simulink model "mrefrobotarm_modified_previous_y_previous_u_previous_ref_pert_2"  (R2018b)
settings: Solver=FixedStepAuto  StartTime=0.0  StopTime=60  RelTol=1e-3  AbsTol=1e-6
undefined symbols (not defined in the file or in its folder): cc, options
libraries: neural x858, simulink x1
(part 20 of 32)

== system mrefrobotarm_modified_previous_y_previous_u_previous_ref_pert_2/m=0 sd=0.3/Layer 3/Delays 1 ==
  "p{3}" : Inport  PortDimensions=30
      mask Display: e = 0.06;c1 = [120 230 180]/255;c2 = ([120 230 180]+0)/(256+128);c3 = ([120 230 180]+128)/(256+128);patch([0 1 1 0],[0 0 1 1],c1);patch([0 1 1 1-e 1-e 0+e],[0 0 1 1-e 0+e 0+e],c2);patch([0 0 1 1-e 0+e 0+e],[0 1 1 1-e 1-e 0+e],c3);plot([0 1 1 0 0],[0 0 1 1 0]);
  mux : Mux  Inputs=1
      mask Display: e = 0.06;c1 = [120 150 230]/255;c2 = ([120 150 230]+0)/383;c3 = ([120 150 230]+128)/383;patch([0 1 1 0],[0 0 1 1],c1);patch([0 1 1 1-e 1-e 0+e],[0 0 1 1-e 0+e 0+e],c2);patch([0 0 1 1-e 0+e 0+e],[0 1 1 1-e 1-e 0+e],c3);plot([0 1 1 0 0],[0 0 1 1 0]);disp('Mux')
  "pd{3,2}" : Outport
      mask Display: e = 0.06;c1 = [120 230 180]/255;c2 = ([120 230 180]+0)/(256+128);c3 = ([120 230 180]+128)/(256+128);patch([0 1 1 0],[0 0 1 1],c1);patch([0 1 1 1-e 1-e 0+e],[0 0 1 1-e 0+e 0+e],c2);patch([0 0 1 1-e 0+e 0+e],[0 1 1 1-e 1-e 0+e],c3);plot([0 1 1 0 0],[0 0 1 1 0]);
  wires:
  "p{3}"/1 -> mux/1
  mux/1 -> "pd{3,2}"/1

== system mrefrobotarm_modified_previous_y_previous_u_previous_ref_pert_2/m=0 sd=0.3/Layer 3/LW{3,2} ==
  "ad{3,2}" : Inport  PortDimensions=30
      mask Display: e = 0.06;c1 = [120 230 180]/255;c2 = ([120 230 180]+0)/(256+128);c3 = ([120 230 180]+128)/(256+128);patch([0 1 1 0],[0 0 1 1],c1);patch([0 1 1 1-e 1-e 0+e],[0 0 1 1-e 0+e 0+e],c2);patch([0 0 1 1-e 0+e 0+e],[0 1 1 1-e 1-e 0+e],c3);plot([0 1 1 0 0],[0 0 1 1 0]);
  "IW{3,2}(1,:)'" : Constant  Value=[0.00073031899760629269587053347123628554982133209705352783203125;0.00015755393865115070316414158657636335192364640533924102783203125;-0.001153726580471188360721424004395885276608169078826904296875;-0.000147810248176156772310918530166645723511464893817901611328125;-0.0003676237953308994737926240770065078322659246623516082763671875;2.047747561014855666172707060468383133411407470703125;-0.000120078654340241940796062125595966563196270726621150970458984375;-0.0001517146347455816213049828444781041980604641139507293701171875;0.001069066277835455623657079371469080797396600246429443359375;-0.000455869268953239151036249676707257094676606357097625732421875;-0.000131416867977301771337750313506376187433488667011260986328125;0.0021027852077354597208624920057218332658521831035614013671875;-0.000428718552194034228930430430182241252623498439788818359375;0.000668702472228331818750179937893562964745797216892242431640625;-0.0002648472831370911047092764345478599352645687758922576904296875;-0.00225575463499039750858710107195292948745191097259521484375;-9.959793829520429873057574265970970373018644750118255615234375e-05;0.00081342038300134486029924207883823328302241861820220947265625;-0.000264647625776768852419451594215615841676481068134307861328125;0.000243069440059264798258131801134140914655290544033050537109375;0.0002546442972532542343457040434628879665979184210300445556640625;-0.000265938721012887375506894560572845875867642462253570556640625;2.880739455805856856908213348145153531731921248137950897216796875e-05;0.0002520358189922171517592663914086870136088691651821136474609375;0.000356179041941332113867246800253951732884161174297332763671875;-0.00126836362647298286389363486392767299548722803592681884765625;-0.00020884518780916460647077703693952344110584817826747894287109375;-0.00105229721959188590556244502494109838153235614299774169921875;0.00416506829530418308527028870003050542436540126800537109375;-0.000261752708499157099066023679512227317900396883487701416015625]
      mask Display: e = 0.06;c1 = [120 150 230]/255;c2 = ([120 150 230]+0)/383;c3 = ([120 150 230]+128)/383;patch([0 1 1 0],[0 0 1 1],c1);patch([0 1 1 1-e 1-e 0+e],[0 0 1 1-e 0+e 0+e],c2);patch([0 0 1 1-e 0+e 0+e],[0 1 1 1-e 1-e 0+e],c3);plot([0 1 1 0 0],[0 0 1 1 0]);disp('weights');
  Mux : Mux  Inputs=1
      mask Display: e = 0.06;c1 = [120 150 230]/255;c2 = ([120 150 230]+0)/383;c3 = ([120 150 230]+128)/383;patch([0 1 1 0],[0 0 1 1],c1);patch([0 1 1 1-e 1-e 0+e],[0 0 1 1-e 0+e 0+e],c2);patch([0 0 1 1-e 0+e 0+e],[0 1 1 1-e 1-e 0+e],c3);plot([0 1 1 0 0],[0 0 1 1 0]);disp('Mux');
  dotprod1 : neural/Weight Functions/dotprod
  "lz{3,2}" : Outport
      mask Display: e = 0.06;c1 = [120 230 180]/255;c2 = ([120 230 180]+0)/(256+128);c3 = ([120 230 180]+128)/(256+128);patch([0 1 1 0],[0 0 1 1],c1);patch([0 1 1 1-e 1-e 0+e],[0 0 1 1-e 0+e 0+e],c2);patch([0 0 1 1-e 0+e 0+e],[0 1 1 1-e 1-e 0+e],c3);plot([0 1 1 0 0],[0 0 1 1 0]);
  wires:
  "IW{3,2}(1,:)'"/1 -> dotprod1/1
  "ad{3,2}"/1 -> dotprod1/2
  dotprod1/1 -> Mux/1
  Mux/1 -> "lz{3,2}"/1

== system mrefrobotarm_modified_previous_y_previous_u_previous_ref_pert_2/m=0 sd=0.4/Layer 1/Delays 1 ==
  "p{1}" : Inport  PortDimensions=10
      mask Display: e = 0.06;c1 = [120 230 180]/255;c2 = ([120 230 180]+0)/(256+128);c3 = ([120 230 180]+128)/(256+128);patch([0 1 1 0],[0 0 1 1],c1);patch([0 1 1 1-e 1-e 0+e],[0 0 1 1-e 0+e 0+e],c2);patch([0 0 1 1-e 0+e 0+e],[0 1 1 1-e 1-e 0+e],c3);plot([0 1 1 0 0],[0 0 1 1 0]);
  mux : Mux  Inputs=1
      mask Display: e = 0.06;c1 = [120 150 230]/255;c2 = ([120 150 230]+0)/383;c3 = ([120 150 230]+128)/383;patch([0 1 1 0],[0 0 1 1],c1);patch([0 1 1 1-e 1-e 0+e],[0 0 1 1-e 0+e 0+e],c2);patch([0 0 1 1-e 0+e 0+e],[0 1 1 1-e 1-e 0+e],c3);plot([0 1 1 0 0],[0 0 1 1 0]);disp('Mux')
  "pd{1,1}" : Outport
      mask Display: e = 0.06;c1 = [120 230 180]/255;c2 = ([120 230 180]+0)/(256+128);c3 = ([120 230 180]+128)/(256+128);patch([0 1 1 0],[0 0 1 1],c1);patch([0 1 1 1-e 1-e 0+e],[0 0 1 1-e 0+e 0+e],c2);patch([0 0 1 1-e 0+e 0+e],[0 1 1 1-e 1-e 0+e],c3);plot([0 1 1 0 0],[0 0 1 1 0]);
  wires:
  "p{1}"/1 -> mux/1
  mux/1 -> "pd{1,1}"/1

== system mrefrobotarm_modified_previous_y_previous_u_previous_ref_pert_2/m=0 sd=0.4/Layer 1/IW{1,1} ==
  "pd{1,1}" : Inport  PortDimensions=10
      mask Display: e = 0.06;c1 = [120 230 180]/255;c2 = ([120 230 180]+0)/(256+128);c3 = ([120 230 180]+128)/(256+128);patch([0 1 1 0],[0 0 1 1],c1);patch([0 1 1 1-e 1-e 0+e],[0 0 1 1-e 0+e 0+e],c2);patch([0 0 1 1-e 0+e 0+e],[0 1 1 1-e 1-e 0+e],c3);plot([0 1 1 0 0],[0 0 1 1 0]);
  "IW{1,1}(1,:)'" : Constant  Value=[4.35535709086524747135626967065036296844482421875;2.42555138809412351719174694153480231761932373046875;-3.131200533605130065240018666372634470462799072265625;-0.5094204285878898286199500944348983466625213623046875;-4.1124371498059364427035689004696905612945556640625;0.51883527624200365124806921812705695629119873046875;6.2562144583090031346728210337460041046142578125;6.60866111511276432821659909677691757678985595703125;-18.935865072294749467118890606798231601715087890625;-15.8212895515813567470786438207142055034637451171875]
      mask Display: e = 0.06;c1 = [120 150 230]/255;c2 = ([120 150 230]+0)/383;c3 = ([120 150 230]+128)/383;patch([0 1 1 0],[0 0 1 1],c1);patch([0 1 1 1-e 1-e 0+e],[0 0 1 1-e 0+e 0+e],c2);patch([0 0 1 1-e 0+e 0+e],[0 1 1 1-e 1-e 0+e],c3);plot([0 1 1 0 0],[0 0 1 1 0]);disp('Weights');
  "IW{1,1}(10,:)'" : Constant  Value=[0.53661031067499298519152262088027782738208770751953125;-1.5017668136177440008083294742391444742679595947265625;0.7806843435083996585177601446048356592655181884765625;-0.04055167714109038368253123962858808226883411407470703125;0.46745642085633065665462027027388103306293487548828125;-0.2664486916861605880768593124230392277240753173828125;-0.46684646576965327380293047099257819354534149169921875;-0.29181588578157813262947684052051045000553131103515625;0.985643356544671167540627720882184803485870361328125;0.50112926067407881358661825288436375558376312255859375]
      mask Display: e = 0.06;c1 = [120 150 230]/255;c2 = ([120 150 230]+0)/383;c3 = ([120 150 230]+128)/383;patch([0 1 1 0],[0 0 1 1],c1);patch([0 1 1 1-e 1-e 0+e],[0 0 1 1-e 0+e 0+e],c2);patch([0 0 1 1-e 0+e 0+e],[0 1 1 1-e 1-e 0+e],c3);plot([0 1 1 0 0],[0 0 1 1 0]);disp('Weights');
  "IW{1,1}(11,:)'" : Constant  Value=[-1.6208798224016811584391462019993923604488372802734375;0.447427977253705144722317754713003523647785186767578125;0.4326080920180384037365683980169706046581268310546875;-0.35807065114767600011447257202235050499439239501953125;0.1833514237293495108271912386044277809560298919677734375;-0.498128112866548067305672020665952004492282867431640625;-0.475650781956347523671269073020084761083126068115234375;-0.46513054714543067280629884407971985638141632080078125;0.65795479078694996122322891096700914204120635986328125;0.25047233937190338526335153801483102142810821533203125]
      mask Display: e = 0.06;c1 = [120 150 230]/255;c2 = ([120 150 230]+0)/383;c3 = ([120 150 230]+128)/383;patch([0 1 1 0],[0 0 1 1],c1);patch([0 1 1 1-e 1-e 0+e],[0 0 1 1-e 0+e 0+e],c2);patch([0 0 1 1-e 0+e 0+e],[0 1 1 1-e 1-e 0+e],c3);plot([0 1 1 0 0],[0 0 1 1 0]);disp('Weights');
  "IW{1,1}(12,:)'" : Constant  Value=[0.89487420700217013003197052967152558267116546630859375;0.0736102811658177202946973238795180805027484893798828125;-0.72097767859178352178872728472924791276454925537109375;0.343010449570382291994974366389214992523193359375;0.05526766853889926445209113126111333258450031280517578125;0.1617754949706347866733580076470389030873775482177734375;-0.09925881285950004240259403331947396509349346160888671875;-0.09491493432806123731193537196304532699286937713623046875;0.266775373828542938792196537178824655711650848388671875;0.296807590311673086258537068715668283402919769287109375]
      mask Display: e = 0.06;c1 = [120 150 230]/255;c2 = ([120 150 230]+0)/383;c3 = ([120 150 230]+128)/383;patch([0 1 1 0],[0 0 1 1],c1);patch([0 1 1 1-e 1-e 0+e],[0 0 1 1-e 0+e 0+e],c2);patch([0 0 1 1-e 0+e 0+e],[0 1 1 1-e 1-e 0+e],c3);plot([0 1 1 0 0],[0 0 1 1 0]);disp('Weights');
  "IW{1,1}(13,:)'" : Constant  Value=[1.0693210911560055986768702496192418038845062255859375;-0.921086541198619546122472456772811710834503173828125;-0.39419926353010570352353170164860785007476806640625;0.6864400832934258733786236916785128414630889892578125;0.13946629961123024887825749829062260687351226806640625;2.8551210111443499073402563226409256458282470703125;-2.673885338519812915336615333217196166515350341796875;-0.434420113181992195716674132199841551482677459716796875;7.617755568501014096227663685567677021026611328125;6.32093063063102977849894159589894115924835205078125]
      mask Display: e = 0.06;c1 = [120 150 230]/255;c2 = ([120 150 230]+0)/383;c3 = ([120 150 230]+128)/383;patch([0 1 1 0],[0 0 1 1],c1);patch([0 1 1 1-e 1-e 0+e],[0 0 1 1-e 0+e 0+e],c2);patch([0 0 1 1-e 0+e 0+e],[0 1 1 1-e 1-e 0+e],c3);plot([0 1 1 0 0],[0 0 1 1 0]);disp('Weights');
  "IW{1,1}(14,:)'" : Constant  Value=[1.58733266996484001509770678239874541759490966796875;-1.9550364500455401639555930159986019134521484375;1.193738170368206841231994985719211399555206298828125;0.1743957236971513113932275018669315613806247711181640625;-0.495270571163230866051918610537541098892688751220703125;0.86398853547281861953166526291170157492160797119140625;0.6502199929278200674076515497290529310703277587890625;0.88327744406018349199172234875732101500034332275390625;-0.7161113464611228440759305158280767500400543212890625;1.1400929339190881695031976050813682377338409423828125]
      mask Display: e = 0.06;c1 = [120 150 230]/255;c2 = ([120 150 230]+0)/383;c3 = ([120 150 230]+128)/383;patch([0 1 1 0],[0 0 1 1],c1);patch([0 1 1 1-e 1-e 0+e],[0 0 1 1-e 0+e 0+e],c2);patch([0 0 1 1-e 0+e 0+e],[0 1 1 1-e 1-e 0+e],c3);plot([0 1 1 0 0],[0 0 1 1 0]);disp('Weights');
  "IW{1,1}(15,:)'" : Constant  Value=[0.45779947364027151479604071937501430511474609375;0.70223579556577020444052550374181009829044342041015625;-0.1281575453302842004799089181688032113015651702880859375;0.12564794902972320489453750269603915512561798095703125;-0.381645372211093292236228080582804977893829345703125;-0.0204190490741921228112776276475415215827524662017822265625;1.0790025966145158076159304982866160571575164794921875;0.287301338557884256008634338286356069147586822509765625;-2.2765111432902305210745907970704138278961181640625;-0.86693087767997401016373260063119232654571533203125]
      mask Display: e = 0.06;c1 = [120 150 230]/255;c2 = ([120 150 230]+0)/383;c3 = ([120 150 230]+128)/383;patch([0 1 1 0],[0 0 1 1],c1);patch([0 1 1 1-e 1-e 0+e],[0 0 1 1-e 0+e 0+e],c2);patch([0 0 1 1-e 0+e 0+e],[0 1 1 1-e 1-e 0+e],c3);plot([0 1 1 0 0],[0 0 1 1 0]);disp('Weights');
  "IW{1,1}(16,:)'" : Constant  Value=[-0.644829761134828149948816644609905779361724853515625;-0.727248367863640776675993038224987685680389404296875;0.642172797313289578369221999309957027435302734375;-0.1544356102039684819349218969364301301538944244384765625;0.61056512859092892941959007657715119421482086181640625;-0.03939013350661614565328960679835290648043155670166015625;-1.547345311753695273893072226201184093952178955078125;-0.9522101260489979068779575754888355731964111328125;3.588158009025375516642952788970433175563812255859375;1.101826384053964602571795694530010223388671875]
      mask Display: e = 0.06;c1 = [120 150 230]/255;c2 = ([120 150 230]+0)/383;c3 = ([120 150 230]+128)/383;patch([0 1 1 0],[0 0 1 1],c1);patch([0 1 1 1-e 1-e 0+e],[0 0 1 1-e 0+e 0+e],c2);patch([0 0 1 1-e 0+e 0+e],[0 1 1 1-e 1-e 0+e],c3);plot([0 1 1 0 0],[0 0 1 1 0]);disp('Weights');
  "IW{1,1}(17,:)'" : Constant  Value=[-0.66194244928404233352381424992927350103855133056640625;-0.2665429905093981144403869620873592793941497802734375;-0.301912534226966566830441252022865228354930877685546875;-0.01267580209757014804428099097322046873159706592559814453125;0.016298170872502480699406390840522362850606441497802734375;0.76567598401868919300028437646687962114810943603515625;-0.5780755859313588818082507714279927313327789306640625;0.61347984886140760618644662827136926352977752685546875;0.82586594226612108915475118919857777655124664306640625;0.357691319136484497942518601121264509856700897216796875]
      mask Display: e = 0.06;c1 = [120 150 230]/255;c2 = ([120 150 230]+0)/383;c3 = ([120 150 230]+128)/383;patch([0 1 1 0],[0 0 1 1],c1);patch([0 1 1 1-e 1-e 0+e],[0 0 1 1-e 0+e 0+e],c2);patch([0 0 1 1-e 0+e 0+e],[0 1 1 1-e 1-e 0+e],c3);plot([0 1 1 0 0],[0 0 1 1 0]);disp('Weights');
  "IW{1,1}(18,:)'" : Constant  Value=[-0.97067823603156100364941494262893684208393096923828125;1.5616920167050414303133720750338397920131683349609375;0.06685278736529849663572377949094516225159168243408203125;0.6499214955341046096037871393491514027118682861328125;-0.262065024340278285297500815431703813374042510986328125;0.3975545099891777400813452914007939398288726806640625;0.60984954015118886250235163970501162111759185791015625;0.017787737644496891264989102410254417918622493743896484375;-0.8088427989736384216001852109911851584911346435546875;0.54858819819970217057658601333969272673130035400390625]
      mask Display: e = 0.06;c1 = [120 150 230]/255;c2 = ([120 150 230]+0)/383;c3 = ([120 150 230]+128)/383;patch([0 1 1 0],[0 0 1 1],c1);patch([0 1 1 1-e 1-e 0+e],[0 0 1 1-e 0+e 0+e],c2);patch([0 0 1 1-e 0+e 0+e],[0 1 1 1-e 1-e 0+e],c3);plot([0 1 1 0 0],[0 0 1 1 0]);disp('Weights');
  "IW{1,1}(19,:)'" : Constant  Value=[0.80345850006630448181255133022204972803592681884765625;0.84832037573162877297505701790214516222476959228515625;1.0509933685202230702060433031874708831310272216796875;-0.29945105490784040824792100465856492519378662109375;0.398413544250740880858785430973512120544910430908203125;-0.62906284888617414186029463962768204510211944580078125;0.419253423393185220557910497518605552613735198974609375;0.1668880001276854263547733125960803590714931488037109375;0.325071746813424600208719539295998401939868927001953125;-0.189742461246484805936773909706971608102321624755859375]
      mask Display: e = 0.06;c1 = [120 150 230]/255;c2 = ([120 150 230]+0)/383;c3 = ([120 150 230]+128)/383;patch([0 1 1 0],[0 0 1 1],c1);patch([0 1 1 1-e 1-e 0+e],[0 0 1 1-e 0+e 0+e],c2);patch([0 0 1 1-e 0+e 0+e],[0 1 1 1-e 1-e 0+e],c3);plot([0 1 1 0 0],[0 0 1 1 0]);disp('Weights');
  "IW{1,1}(2,:)'" : Constant  Value=[-0.069682631558683649775076673904550261795520782470703125;-0.1639974482889220708248245728100300766527652740478515625;0.12283683760710613352973297196513158269226551055908203125;-0.4808737441971653314709556070738472044467926025390625;0.1034846041578211528477737601861008442938327789306640625;-0.525225386921444936660918756388127803802490234375;-0.393646581016063923375014610428479500114917755126953125;-0.64042997244119359567804394828272052109241485595703125;0.030514809530166435436182581497632781974971294403076171875;-0.56273534850692008557615508834715001285076141357421875]
      mask Display: e = 0.06;c1 = [120 150 230]/255;c2 = ([120 150 230]+0)/383;c3 = ([120 150 230]+128)/383;patch([0 1 1 0],[0 0 1 1],c1);patch([0 1 1 1-e 1-e 0+e],[0 0 1 1-e 0+e 0+e],c2);patch([0 0 1 1-e 0+e 0+e],[0 1 1 1-e 1-e 0+e],c3);plot([0 1 1 0 0],[0 0 1 1 0]);disp('Weights');
  "IW{1,1}(20,:)'" : Constant  Value=[-0.4107285391497583759701228700578212738037109375;1.408803689080053711535356342210434377193450927734375;0.451929861878933747387776520554325543344020843505859375;0.00479686782901274540169556104274306562729179859161376953125;0.24357580890878949286815213781665079295635223388671875;0.12049863564349073963288816457861685194075107574462890625;0.88810099930725616701465696678496897220611572265625;0.8037487613823321996875392869696952402591705322265625;-0.82572616695100797823414495724136941134929656982421875;-1.0830952787283616434166333419852890074253082275390625]
      mask Display: e = 0.06;c1 = [120 150 230]/255;c2 = ([120 150 230]+0)/383;c3 = ([120 150 230]+128)/383;patch([0 1 1 0],[0 0 1 1],c1);patch([0 1 1 1-e 1-e 0+e],[0 0 1 1-e 0+e 0+e],c2);patch([0 0 1 1-e 0+e 0+e],[0 1 1 1-e 1-e 0+e],c3);plot([0 1 1 0 0],[0 0 1 1 0]);disp('Weights');
  "IW{1,1}(21,:)'" : Constant  Value=[0.423864698803549211358898674006923101842403411865234375;0.33451003427855929839296322825248353183269500732421875;-0.1233720521424563620893621873619849793612957000732421875;0.00362782141401441805828032016734141507185995578765869140625;-0.072209282480322711794684664710075594484806060791015625;-0.40856050052729242505478168823174200952053070068359375;0.385969239676839992458923234153189696371555328369140625;-0.12455233740777553463896509811092982999980449676513671875;-0.0441511799769076784816235203834366984665393829345703125;-0.23944975493487363760181096949963830411434173583984375]
      mask Display: e = 0.06;c1 = [120 150 230]/255;c2 = ([120 150 230]+0)/383;c3 = ([120 150 230]+128)/383;patch([0 1 1 0],[0 0 1 1],c1);patch([0 1 1 1-e 1-e 0+e],[0 0 1 1-e 0+e 0+e],c2);patch([0 0 1 1-e 0+e 0+e],[0 1 1 1-e 1-e 0+e],c3);plot([0 1 1 0 0],[0 0 1 1 0]);disp('Weights');
  "IW{1,1}(22,:)'" : Constant  Value=[0.0803218316576901347758621341199614107608795166015625;0.0328619355980256655502813600833178497850894927978515625;-0.17962704900125725515636077034287154674530029296875;-0.1215825658357615746130164779970073141157627105712890625;-0.60019397848763678116057462830212898552417755126953125;0.21629668123979783889154759890516288578510284423828125;0.0111474316272483463252651603170306771062314510345458984375;-0.1571384847164933040719603241086588241159915924072265625;-1.6394482078873888752923448919318616390228271484375;-0.5111554971429497218338156017125584185123443603515625]
      mask Display: e = 0.06;c1 = [120 150 230]/255;c2 = ([120 150 230]+0)/383;c3 = ([120 150 230]+128)/383;patch([0 1 1 0],[0 0 1 1],c1);patch([0 1 1 1-e 1-e 0+e],[0 0 1 1-e 0+e 0+e],c2);patch([0 0 1 1-e 0+e 0+e],[0 1 1 1-e 1-e 0+e],c3);plot([0 1 1 0 0],[0 0 1 1 0]);disp('Weights');
  "IW{1,1}(23,:)'" : Constant  Value=[1.5795529317278791392453740627388469874858856201171875;-0.85097215011614724122779307435848750174045562744140625;-0.327361229627383620854885748485685326159000396728515625;0.06749982790787113773323113719015964306890964508056640625;-0.12385644995348944752411313174889073707163333892822265625;-0.876452542132245771000498280045576393604278564453125;0.9860297613247428483163048440474085509777069091796875;0.25843472744673601226850223611108958721160888671875;-2.3417502384200883369658185984008014202117919921875;-1.9110154646430708158533207097207196056842803955078125]
      mask Display: e = 0.06;c1 = [120 150 230]/255;c2 = ([120 150 230]+0)/383;c3 = ([120 150 230]+128)/383;patch([0 1 1 0],[0 0 1 1],c1);patch([0 1 1 1-e 1-e 0+e],[0 0 1 1-e 0+e 0+e],c2);patch([0 0 1 1-e 0+e 0+e],[0 1 1 1-e 1-e 0+e],c3);plot([0 1 1 0 0],[0 0 1 1 0]);disp('Weights');
  "IW{1,1}(24,:)'" : Constant  Value=[-0.273608247375458246697377262535155750811100006103515625;-1.38744487071924549326240594382397830486297607421875;0.96428753975518244345721541321836411952972412109375;0.446109064592351500788680596087942831218242645263671875;-0.343565458378224997115779615342034958302974700927734375;0.141572622071520604070116178263560868799686431884765625;-0.10303621291445852481416523005464114248752593994140625;-0.2179509085022676428966548201060504652559757232666015625;-1.434288374880912986242265105829574167728424072265625;-0.451422810908673588503603468780056573450565338134765625]
      mask Display: e = 0.06;c1 = [120 150 230]/255;c2 = ([120 150 230]+0)/383;c3 = ([120 150 230]+128)/383;patch([0 1 1 0],[0 0 1 1],c1);patch([0 1 1 1-e 1-e 0+e],[0 0 1 1-e 0+e 0+e],c2);patch([0 0 1 1-e 0+e 0+e],[0 1 1 1-e 1-e 0+e],c3);plot([0 1 1 0 0],[0 0 1 1 0]);disp('Weights');
  "IW{1,1}(25,:)'" : Constant  Value=[-1.149162177122760919445454419474117457866668701171875;0.1086860018629928481548319041394279338419437408447265625;0.266344644983039058327989323515794239938259124755859375;-0.070024145185166364324658161422121338546276092529296875;-0.270922740810928652788192039224668405950069427490234375;-0.127408901597892365575859230375499464571475982666015625;-0.48942693267029280246305233958992175757884979248046875;-0.042249209130051278149320381771758547984063625335693359375;-0.651907282090750328507056110538542270660400390625;-0.95647767621304102814150382982916198670864105224609375]
      mask Display: e = 0.06;c1 = [120 150 230]/255;c2 = ([120 150 230]+0)/383;c3 = ([120 150 230]+128)/383;patch([0 1 1 0],[0 0 1 1],c1);patch([0 1 1 1-e 1-e 0+e],[0 0 1 1-e 0+e 0+e],c2);patch([0 0 1 1-e 0+e 0+e],[0 1 1 1-e 1-e 0+e],c3);plot([0 1 1 0 0],[0 0 1 1 0]);disp('Weights');
  "IW{1,1}(26,:)'" : Constant  Value=[-1.165319098111982309973200244712643325328826904296875;0.72145939551326898619976191184832714498043060302734375;-0.90522219406142967468298365929513238370418548583984375;0.447571892827514694612744960977579466998577117919921875;0.29342760953863444850497899096808396279811859130859375;-1.5440447426337164937848456247593276202678680419921875;0.29317133111777227139072010686504654586315155029296875;-1.275932731387730001415548031218349933624267578125;-2.302051195328274513229871445219032466411590576171875;-3.271613930691695149022280020290054380893707275390625]
      mask Display: e = 0.06;c1 = [120 150 230]/255;c2 = ([120 150 230]+0)/383;c3 = ([120 150 230]+128)/383;patch([0 1 1 0],[0 0 1 1],c1);patch([0 1 1 1-e 1-e 0+e],[0 0 1 1-e 0+e 0+e],c2);patch([0 0 1 1-e 0+e 0+e],[0 1 1 1-e 1-e 0+e],c3);plot([0 1 1 0 0],[0 0 1 1 0]);disp('Weights');
  "IW{1,1}(27,:)'" : Constant  Value=[0.7494377068539639363820015205419622361660003662109375;-2.0777830408087165636743520735763013362884521484375;0.647415456446395864986698143184185028076171875;1.022306436395755024904019592213444411754608154296875;-1.2371930913673525598284186344244517385959625244140625;-0.135042762815553663013901086742407642304897308349609375;1.2622513327665150217882228389498777687549591064453125;-0.39147255740735775741967472640681080520153045654296875;-1.35141904515557254029545219964347779750823974609375;-1.1604605296168684080981847728253342211246490478515625]
      mask Display: e = 0.06;c1 = [120 150 230]/255;c2 = ([120 150 230]+0)/383;c3 = ([120 150 230]+128)/383;patch([0 1 1 0],[0 0 1 1],c1);patch([0 1 1 1-e 1-e 0+e],[0 0 1 1-e 0+e 0+e],c2);patch([0 0 1 1-e 0+e 0+e],[0 1 1 1-e 1-e 0+e],c3);plot([0 1 1 0 0],[0 0 1 1 0]);disp('Weights');
  "IW{1,1}(28,:)'" : Constant  Value=[-1.5104734553801966168151693636900745332241058349609375;1.6562503399973433904079911371809430420398712158203125;-0.472067614297997817374152873526327311992645263671875;-0.05048243394340622136606810954617685638368129730224609375;0.52372481749565824582504092177259735763072967529296875;1.19295218648003409356306292465887963771820068359375;-0.861776283455968350466491756378673017024993896484375;-1.58684696306389039222040082677267491817474365234375;2.257509580845225460876690704026259481906890869140625;3.41542439317276613763851855765096843242645263671875]
      mask Display: e = 0.06;c1 = [120 150 230]/255;c2 = ([120 150 230]+0)/383;c3 = ([120 150 230]+128)/383;patch([0 1 1 0],[0 0 1 1],c1);patch([0 1 1 1-e 1-e 0+e],[0 0 1 1-e 0+e 0+e],c2);patch([0 0 1 1-e 0+e 0+e],[0 1 1 1-e 1-e 0+e],c3);plot([0 1 1 0 0],[0 0 1 1 0]);disp('Weights');
  "IW{1,1}(29,:)'" : Constant  Value=[0.4690028791331286583954351954162120819091796875;-0.2783012675515834644102142192423343658447265625;-0.07854654990007668702300946961258887313306331634521484375;-0.07898553729212030860562521183965145610272884368896484375;0.46624959546653688136075288639403879642486572265625;-0.2080655768261337745794747888794518075883388519287109375;-0.257523219663172486804114669212140142917633056640625;0.08794913971768902882786278496496379375457763671875;1.6718270736216032101850714752799831330776214599609375;0.4081716567304678466854284124565310776233673095703125]
      mask Display: e = 0.06;c1 = [120 150 230]/255;c2 = ([120 150 230]+0)/383;c3 = ([120 150 230]+128)/383;patch([0 1 1 0],[0 0 1 1],c1);patch([0 1 1 1-e 1-e 0+e],[0 0 1 1-e 0+e 0+e],c2);patch([0 0 1 1-e 0+e 0+e],[0 1 1 1-e 1-e 0+e],c3);plot([0 1 1 0 0],[0 0 1 1 0]);disp('Weights');
  "IW{1,1}(3,:)'" : Constant  Value=[-0.05465814106178555620285663962931721471250057220458984375;0.0549728918272474886830281093352823518216609954833984375;0.0179710362373937775071208733379535260610282421112060546875;0.021276513140936537116232329935883171856403350830078125;0.08930177865023654348863857421747525222599506378173828125;-0.03788970242810872635086383297675638459622859954833984375;-0.018492973827131164998860413106740452349185943603515625;0.03816879199061039285023611000724486075341701507568359375;0.313698522894576503627916963523603044450283050537109375;0.0778393180610279511455473766545765101909637451171875]
      mask Display: e = 0.06;c1 = [120 150 230]/255;c2 = ([120 150 230]+0)/383;c3 = ([120 150 230]+128)/383;patch([0 1 1 0],[0 0 1 1],c1);patch([0 1 1 1-e 1-e 0+e],[0 0 1 1-e 0+e 0+e],c2);patch([0 0 1 1-e 0+e 0+e],[0 1 1 1-e 1-e 0+e],c3);plot([0 1 1 0 0],[0 0 1 1 0]);disp('Weights');
  "IW{1,1}(30,:)'" : Constant  Value=[0.1375770100337117274325038351889816112816333770751953125;-0.53921863271993364374878865419304929673671722412109375;0.165527397854886293426801557870930992066860198974609375;-0.1699060332404046802512453950839699245989322662353515625;0.179938472485099920650242211195291019976139068603515625;-0.52592447692005972470496999449096620082855224609375;0.1369154139480974474718522060356917791068553924560546875;-0.40446546294877416816149207079433836042881011962890625;-0.69691858462240230398521134702605195343494415283203125;-0.62819206434997543198051062063314020633697509765625]
      mask Display: e = 0.06;c1 = [120 150 230]/255;c2 = ([120 150 230]+0)/383;c3 = ([120 150 230]+128)/383;patch([0 1 1 0],[0 0 1 1],c1);patch([0 1 1 1-e 1-e 0+e],[0 0 1 1-e 0+e 0+e],c2);patch([0 0 1 1-e 0+e 0+e],[0 1 1 1-e 1-e 0+e],c3);plot([0 1 1 0 0],[0 0 1 1 0]);disp('Weights');
  "IW{1,1}(4,:)'" : Constant  Value=[0.08043726636398733365052038379872101359069347381591796875;-0.68708545467906734227625520361470989882946014404296875;0.345743421716964538514815785674727521836757659912109375;-0.6423919698675870648685304331593215465545654296875;0.0602499264563745862144372722468688152730464935302734375;-0.316987201527190787242460601191851310431957244873046875;-0.2341436713578660400170150523990741930902004241943359375;0.003845871605578733698482807312757358886301517486572265625;0.02888157472152076687965660539703094400465488433837890625;-0.394414468880340318701627211339655332267284393310546875]
      mask Display: e = 0.06;c1 = [120 150 230]/255;c2 = ([120 150 230]+0)/383;c3 = ([120 150 230]+128)/383;patch([0 1 1 0],[0 0 1 1],c1);patch([0 1 1 1-e 1-e 0+e],[0 0 1 1-e 0+e 0+e],c2);patch([0 0 1 1-e 0+e 0+e],[0 1 1 1-e 1-e 0+e],c3);plot([0 1 1 0 0],[0 0 1 1 0]);disp('Weights');
  "IW{1,1}(5,:)'" : Constant  Value=[-0.6861604686211124626282753524719737470149993896484375;-0.112219277728957955719835126728867180645465850830078125;0.64917860399719218289504851782112382352352142333984375;-0.6037971691378007932371474453248083591461181640625;-0.06351370453928097126183871523608104325830936431884765625;-0.75880872040184554894182156203896738588809967041015625;0.369525119529071910395856548348092474043369293212890625;0.4130281829261530646135724964551627635955810546875;-1.8220859535603912693346728701726533472537994384765625;-1.9857637080258336848004319108440540730953216552734375]
      mask Display: e = 0.06;c1 = [120 150 230]/255;c2 = ([120 150 230]+0)/383;c3 = ([120 150 230]+128)/383;patch([0 1 1 0],[0 0 1 1],c1);patch([0 1 1 1-e 1-e 0+e],[0 0 1 1-e 0+e 0+e],c2);patch([0 0 1 1-e 0+e 0+e],[0 1 1 1-e 1-e 0+e],c3);plot([0 1 1 0 0],[0 0 1 1 0]);disp('Weights');
  "IW{1,1}(6,:)'" : Constant  Value=[0.45886514466681227464306402907823212444782257080078125;-0.11142595798238179305439388144804979674518108367919921875;-0.42504318155345455210181171423755586147308349609375;-0.934139409727496872193341914680786430835723876953125;0.303864171931082671651580540128634311258792877197265625;0.51465097566426531994210336051764898002147674560546875;-0.9717551642348369878021685508429072797298431396484375;0.03663383154416273435050044326999341137707233428955078125;2.836510990175402202595478229341097176074981689453125;1.7540319866470632792498918206547386944293975830078125]
      mask Display: e = 0.06;c1 = [120 150 230]/255;c2 = ([120 150 230]+0)/383;c3 = ([120 150 230]+128)/383;patch([0 1 1 0],[0 0 1 1],c1);patch([0 1 1 1-e 1-e 0+e],[0 0 1 1-e 0+e 0+e],c2);patch([0 0 1 1-e 0+e 0+e],[0 1 1 1-e 1-e 0+e],c3);plot([0 1 1 0 0],[0 0 1 1 0]);disp('Weights');
  "IW{1,1}(7,:)'" : Constant  Value=[-0.1586306098935577335584667935108882375061511993408203125;0.2395721967577284783335045403873664326965808868408203125;-0.08727907337821354250007033215297269634902477264404296875;0.500328613778542763412815475021488964557647705078125;-0.1097938134199833715154426272420096211135387420654296875;-0.8215419198343869577882969679194502532482147216796875;0.6440357126179760971496079946518875658512115478515625;0.052916979193343573195651430296493344940245151519775390625;-0.591804462003254538871033219038508832454681396484375;-0.380004215885382190531771584574016742408275604248046875]
      mask Display: e = 0.06;c1 = [120 150 230]/255;c2 = ([120 150 230]+0)/383;c3 = ([120 150 230]+128)/383;patch([0 1 1 0],[0 0 1 1],c1);patch([0 1 1 1-e 1-e 0+e],[0 0 1 1-e 0+e 0+e],c2);patch([0 0 1 1-e 0+e 0+e],[0 1 1 1-e 1-e 0+e],c3);plot([0 1 1 0 0],[0 0 1 1 0]);disp('Weights');
  "IW{1,1}(8,:)'" : Constant  Value=[0.1654933157640761098861048594699241220951080322265625;-0.16425950115592169442635395171237178146839141845703125;-0.1730383341514245554293438544846139848232269287109375;-0.07190829145436135327873472533610765822231769561767578125;-0.03550222626676548254298637630199664272367954254150390625;-0.1216959832574034672258989075999124906957149505615234375;0.00261606307143610015975010441025006002746522426605224609375;-0.2146907369188607306309535260879783891141414642333984375;-0.6112389006926537415864686408895067870616912841796875;-0.278758616809984260953569901175796985626220703125]
      mask Display: e = 0.06;c1 = [120 150 230]/255;c2 = ([120 150 230]+0)/383;c3 = ([120 150 230]+128)/383;patch([0 1 1 0],[0 0 1 1],c1);patch([0 1 1 1-e 1-e 0+e],[0 0 1 1-e 0+e 0+e],c2);patch([0 0 1 1-e 0+e 0+e],[0 1 1 1-e 1-e 0+e],c3);plot([0 1 1 0 0],[0 0 1 1 0]);disp('Weights');
  "IW{1,1}(9,:)'" : Constant  Value=[0.03337126303870606436330348287810920737683773040771484375;-0.369217929731265381843030581876519136130809783935546875;-0.13449767564821868415236849614302627742290496826171875;0.4454375651864257434908722643740475177764892578125;0.35525518068719541542321849192376248538494110107421875;-1.5423744058518444877137199000571854412555694580078125;0.842618792986030484826187603175640106201171875;-0.02454352513655795597902198323936318047344684600830078125;-2.248953263110823996839826577343046665191650390625;-2.381855622416273465802305508987046778202056884765625]
      mask Display: e = 0.06;c1 = [120 150 230]/255;c2 = ([120 150 230]+0)/383;c3 = ([120 150 230]+128)/383;patch([0 1 1 0],[0 0 1 1],c1);patch([0 1 1 1-e 1-e 0+e],[0 0 1 1-e 0+e 0+e],c2);patch([0 0 1 1-e 0+e 0+e],[0 1 1 1-e 1-e 0+e],c3);plot([0 1 1 0 0],[0 0 1 1 0]);disp('Weights');
  Mux : Mux  Inputs=30
      mask Display: e = 0.06;c1 = [120 150 230]/255;c2 = ([120 150 230]+0)/383;c3 = ([120 150 230]+128)/383;patch([0 1 1 0],[0 0 1 1],c1);patch([0 1 1 1-e 1-e 0+e],[0 0 1 1-e 0+e 0+e],c2);patch([0 0 1 1-e 0+e 0+e],[0 1 1 1-e 1-e 0+e],c3);plot([0 1 1 0 0],[0 0 1 1 0]);disp('Mux');
  dotprod{1..30} (30 alike) : neural/Weight Functions/dotprod
  "iz{1,1}" : Outport
      mask Display: e = 0.06;c1 = [120 230 180]/255;c2 = ([120 230 180]+0)/(256+128);c3 = ([120 230 180]+128)/(256+128);patch([0 1 1 0],[0 0 1 1],c1);patch([0 1 1 1-e 1-e 0+e],[0 0 1 1-e 0+e 0+e],c2);patch([0 0 1 1-e 0+e 0+e],[0 1 1 1-e 1-e 0+e],c3);plot([0 1 1 0 0],[0 0 1 1 0]);
  wires:
  "IW{1,1}(1,:)'"/1 -> dotprod1/1
  "pd{1,1}"/1 -> dotprod1/2, dotprod2/2, dotprod3/2, dotprod4/2, dotprod5/2, dotprod6/2, dotprod7/2, dotprod8/2, dotprod9/2, dotprod10/2, dotprod11/2, dotprod12/2, dotprod13/2, dotprod14/2, dotprod15/2, dotprod16/2, dotprod17/2, dotprod18/2, dotprod19/2, dotprod20/2, dotprod21/2, dotprod22/2, dotprod23/2, dotprod24/2, dotprod25/2, dotprod26/2, dotprod27/2, dotprod28/2, dotprod29/2, dotprod30/2
  dotprod1/1 -> Mux/1
  "IW{1,1}(2,:)'"/1 -> dotprod2/1
  dotprod2/1 -> Mux/2
  "IW{1,1}(3,:)'"/1 -> dotprod3/1
  dotprod3/1 -> Mux/3
  "IW{1,1}(4,:)'"/1 -> dotprod4/1
  dotprod4/1 -> Mux/4
  "IW{1,1}(5,:)'"/1 -> dotprod5/1
  dotprod5/1 -> Mux/5
  "IW{1,1}(6,:)'"/1 -> dotprod6/1
  dotprod6/1 -> Mux/6
  "IW{1,1}(7,:)'"/1 -> dotprod7/1
  dotprod7/1 -> Mux/7
  "IW{1,1}(8,:)'"/1 -> dotprod8/1
  dotprod8/1 -> Mux/8
  "IW{1,1}(9,:)'"/1 -> dotprod9/1
  dotprod9/1 -> Mux/9
  "IW{1,1}(10,:)'"/1 -> dotprod10/1
  dotprod10/1 -> Mux/10
  "IW{1,1}(11,:)'"/1 -> dotprod11/1
  dotprod11/1 -> Mux/11
  "IW{1,1}(12,:)'"/1 -> dotprod12/1
  dotprod12/1 -> Mux/12
  "IW{1,1}(13,:)'"/1 -> dotprod13/1
  dotprod13/1 -> Mux/13
  "IW{1,1}(14,:)'"/1 -> dotprod14/1
  dotprod14/1 -> Mux/14
  "IW{1,1}(15,:)'"/1 -> dotprod15/1
  dotprod15/1 -> Mux/15
  "IW{1,1}(16,:)'"/1 -> dotprod16/1
  dotprod16/1 -> Mux/16
  "IW{1,1}(17,:)'"/1 -> dotprod17/1
  dotprod17/1 -> Mux/17
  "IW{1,1}(18,:)'"/1 -> dotprod18/1
  dotprod18/1 -> Mux/18
  "IW{1,1}(19,:)'"/1 -> dotprod19/1
  dotprod19/1 -> Mux/19
  "IW{1,1}(20,:)'"/1 -> dotprod20/1
  dotprod20/1 -> Mux/20
  "IW{1,1}(21,:)'"/1 -> dotprod21/1
  dotprod21/1 -> Mux/21
  "IW{1,1}(22,:)'"/1 -> dotprod22/1
  dotprod22/1 -> Mux/22
  "IW{1,1}(23,:)'"/1 -> dotprod23/1
  dotprod23/1 -> Mux/23
  "IW{1,1}(24,:)'"/1 -> dotprod24/1
  dotprod24/1 -> Mux/24
  "IW{1,1}(25,:)'"/1 -> dotprod25/1
  dotprod25/1 -> Mux/25
  "IW{1,1}(26,:)'"/1 -> dotprod26/1
  dotprod26/1 -> Mux/26
  "IW{1,1}(27,:)'"/1 -> dotprod27/1
  dotprod27/1 -> Mux/27
  "IW{1,1}(28,:)'"/1 -> dotprod28/1
  dotprod28/1 -> Mux/28
  "IW{1,1}(29,:)'"/1 -> dotprod29/1
  dotprod29/1 -> Mux/29
  "IW{1,1}(30,:)'"/1 -> dotprod30/1
  dotprod30/1 -> Mux/30
  Mux/1 -> "iz{1,1}"/1

== system mrefrobotarm_modified_previous_y_previous_u_previous_ref_pert_2/m=0 sd=0.4/Layer 2/Delays 1 ==
  "p{2}" : Inport  PortDimensions=30
      mask Display: e = 0.06;c1 = [120 230 180]/255;c2 = ([120 230 180]+0)/(256+128);c3 = ([120 230 180]+128)/(256+128);patch([0 1 1 0],[0 0 1 1],c1);patch([0 1 1 1-e 1-e 0+e],[0 0 1 1-e 0+e 0+e],c2);patch([0 0 1 1-e 0+e 0+e],[0 1 1 1-e 1-e 0+e],c3);plot([0 1 1 0 0],[0 0 1 1 0]);
  mux : Mux  Inputs=1
      mask Display: e = 0.06;c1 = [120 150 230]/255;c2 = ([120 150 230]+0)/383;c3 = ([120 150 230]+128)/383;patch([0 1 1 0],[0 0 1 1],c1);patch([0 1 1 1-e 1-e 0+e],[0 0 1 1-e 0+e 0+e],c2);patch([0 0 1 1-e 0+e 0+e],[0 1 1 1-e 1-e 0+e],c3);plot([0 1 1 0 0],[0 0 1 1 0]);disp('Mux')
  "pd{2,1}" : Outport
      mask Display: e = 0.06;c1 = [120 230 180]/255;c2 = ([120 230 180]+0)/(256+128);c3 = ([120 230 180]+128)/(256+128);patch([0 1 1 0],[0 0 1 1],c1);patch([0 1 1 1-e 1-e 0+e],[0 0 1 1-e 0+e 0+e],c2);patch([0 0 1 1-e 0+e 0+e],[0 1 1 1-e 1-e 0+e],c3);plot([0 1 1 0 0],[0 0 1 1 0]);
  wires:
  "p{2}"/1 -> mux/1
  mux/1 -> "pd{2,1}"/1
